simulink model "simModel"  (R2020a)
settings: Solver=VariableStepAuto  StartTime=0.0  StopTime=Simulation_Time  RelTol=1e-3
InitFcn:
  | ks = 500.4;
  | bs = 24.67;
  | 
  | ms = 325;               % 1/4 sprung mass (kg)
  | mus = 65;               % 1/4 unsprung mass (kg)
  | kus = 500.5e2;          % tire stiffness (N/m)
  | bus = 0;
  | grav = 9.81;            % acceleration of gravity (m/s^2)
  | v = 10;                 % vehicle velocity (m/s)
  | ts = 0.05;             % sampling time step
  | 
  | % Construct linear state space model
  | Aqcar = [-bs/ms -ks/ms bs/ms ks/ms;  1 0  0 0; bs/mus ks/mus -(bs+bus)/mus -(ks+kus)/mus; 0 0 1 0];
  | Bqcar = [1/ms 0 -1/mus 0;0 0 kus/mus 0]';
  | Cqcar = eye(4);
  | Dqcar = zeros(2,4)';
StopFcn:
  | clear ks bs  ms mus kus bus Aqcar Bqcar Cqcar Dqcar
values from neighbouring files (symbols this model uses):
  A = J    [CalculateMPC.m]    (also in CalculateMPC_IMP.m; Plant_Model.m = [ 0 0 1 0; returnStateSpace.m = [0 0 1 0)
  Aq = (eye(dimA)+A*T)    [FORWARDEULER.m]    (also in Get_Model_Script.m = [RP1.Data(end,[1:4]); Plant_Model_ZOH.m = sys.A)
  B = [0 0 ... (first row only)    [Plant_Model.m]    (also in returnStateSpace.m = [ 0 0 0)
  Bq = B*T    [FORWARDEULER.m]    (also in Get_Model_Script.m = [RP1.Data(end,[5:7]); Plant_Model_ZOH.m = sys.B)
  C = [-1 1 0 0 ... (first row only)    [Plant_Model.m]    (also in returnStateSpace.m)
  Cq = C    [FORWARDEULER.m]    (also in Plant_Model_ZOH.m = sys.C)
  D = [0 0;0 0; 0 -1; 0 0]    [Plant_Model.m]    (also in returnStateSpace.m = [0 0 0)
  Dq = D    [FORWARDEULER.m]    (also in Plant_Model_ZOH.m = sys.D)
  FILTER = 20    [BasicLeastSquares7.m]    (also in Get_Model_Script.m = 99999)
  NOISE = 0.00    (= 0)    [BasicLeastSquares7.m]    (also in BasicLeastSquares7_orig.m; CalculateMPC.m = 0.05; CalculateMPC_IMP.m = 0.05; Get_Model_Script.m = 0.05)
  SEED = 100    [Get_Model_Script.m]
  Simulation_Time = (points)*T    (= 100)    [BasicLeastSquares7.m]    (also in BasicLeastSquares7_orig.m = 10; Get_Model_Script.m = 500)
  T = 0.1    [BasicLeastSquares7.m]    (also in BasicLeastSquares7_orig.m = 0.0001; CalculateMPC.m = 0.05; CalculateMPC_IMP.m = 0.05; Get_Model_Script.m = 0.05)
libraries: simulink x7, cstblocks x1
PauseFcn:
  | clear ks bs  ms mus bus kus Aqcar Bqcar Cqcar Dqcar
settings Model: TunableVars=ts  TunableVarsStorageClass=Auto  Creator=manziec  LastModifiedBy=jakelangton
settings DataIOCC: SaveOutput=off  SaveTime=off  ReturnWorkspaceOutputs=off
settings OptimizationCC: DefaultParameterBehavior=Inlined
settings DebuggingCC: ArithmeticOperatorsInVariantConditions=warning
settings SFSimCC: CustomCodeUndefinedFunction=UseInterfaceOnly

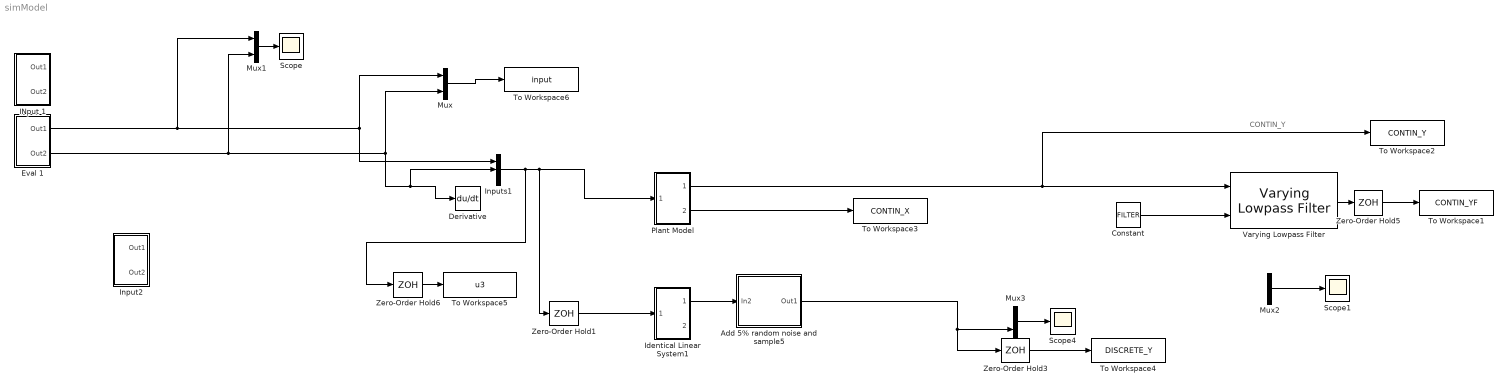
== system simModel ==
  note: CONTIN_Y
  Add 5% random noise and sample5 : Subsystem
  Constant : Constant  Value=FILTER
  Derivative : Derivative
  Eval 1 : Subsystem
  INput 1 : Subsystem
  Identical Linear System1 : Subsystem
  Input2 : Subsystem
  Inputs1 : Mux  Inputs=3
  Mux{,1..3} (4 alike) : Mux  Inputs=2
  Plant Model : Subsystem
  Scope : Scope
  Scope1 : Scope
  Scope4 : Scope
  To Workspace1 : ToWorkspace  VariableName=CONTIN_YF  SaveFormat=Timeseries  SampleTime=-1
  To Workspace2 : ToWorkspace  VariableName=CONTIN_Y  SaveFormat=Timeseries  SampleTime=-1
  To Workspace3 : ToWorkspace  VariableName=CONTIN_X  SaveFormat=Timeseries  SampleTime=-1
  To Workspace4 : ToWorkspace  VariableName=DISCRETE_Y  SaveFormat=Timeseries  SampleTime=-1
  To Workspace5 : ToWorkspace  VariableName=u3  SaveFormat=Timeseries  SampleTime=-1
  To Workspace6 : ToWorkspace  VariableName=input  SaveFormat=Timeseries  SampleTime=-1
  Varying Lowpass Filter : cstblocks/Linear Parameter Varying/Varying Lowpass Filter  N=1
  Zero-Order Hold{1,3,5..6} (4 alike) : ZeroOrderHold  SampleTime=T
  wires:
  Mux3/1 -> Scope4/1
  Inputs1/1 -> Zero-Order Hold6/1, Plant Model/1(In1), Zero-Order Hold1/1
  Add 5% random noise and sample5/1(Out1) -> Zero-Order Hold3/1, Mux3/2
  Identical Linear System1/1(Out1) -> Add 5% random noise and sample5/1(In2)
  Zero-Order Hold3/1 -> To Workspace4/1
  Zero-Order Hold6/1 -> To Workspace5/1
  Mux2/1 -> Scope1/1
  Zero-Order Hold1/1 -> Identical Linear System1/1(In1)
  Constant/1 -> Varying Lowpass Filter/2
  Zero-Order Hold5/1 -> To Workspace1/1
  Varying Lowpass Filter/1 -> Zero-Order Hold5/1
  Plant Model/1(Out1) -> To Workspace2/1, Varying Lowpass Filter/1
  Plant Model/2(Out2) -> To Workspace3/1
  Mux/1 -> To Workspace6/1
  Eval 1/2(Out2) -> Mux1/2, Derivative/1, Inputs1/2, Mux/2
  Mux1/1 -> Scope/1
  Eval 1/1(Out1) -> Mux1/1, Mux/1, Inputs1/1

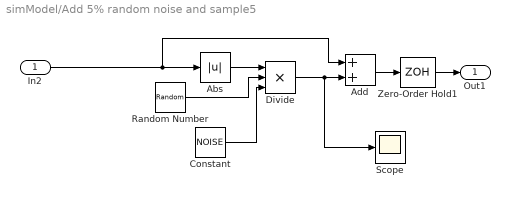
== system simModel/Add 5% random noise and sample5 ==
  In2 : Inport
  Abs : Abs
  Add : Sum
  Constant : Constant  Value=NOISE
  Divide : Product  Inputs=***
  Random Number : RandomNumber  Seed=123  SampleTime=T/10
  Scope : Scope
  Zero-Order Hold1 : ZeroOrderHold  SampleTime=T/10
  Out1 : Outport  VectorParamsAs1DForOutWhenUnconnected=off
  wires:
  Add/1 -> Zero-Order Hold1/1
  Zero-Order Hold1/1 -> Out1/1
  Random Number/1 -> Divide/2
  Abs/1 -> Divide/1
  In2/1 -> Abs/1, Add/1
  Constant/1 -> Divide/3
  Divide/1 -> Add/2, Scope/1

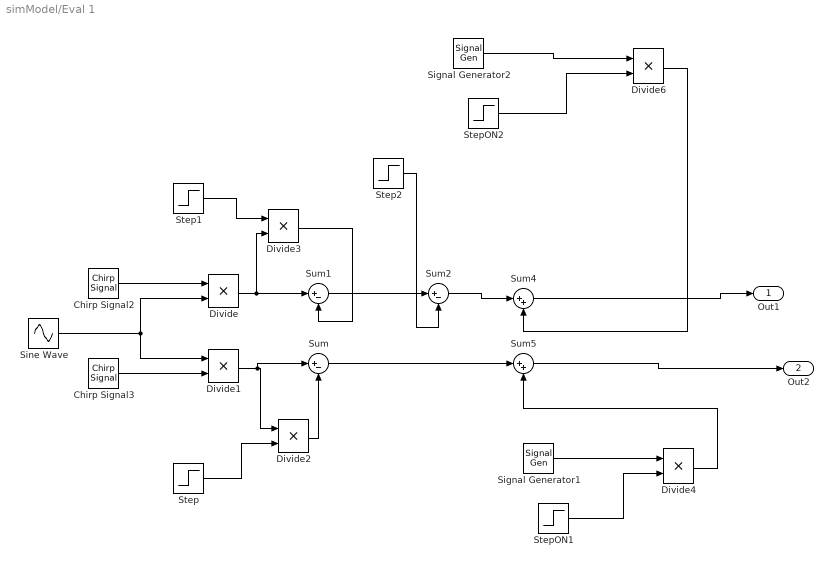
== system simModel/Eval 1 ==
  Chirp Signal2 : simulink/Sources/Chirp Signal  f1=0.01  T=Simulation_Time*3/4  f2=10
  Chirp Signal3 : simulink/Sources/Chirp Signal  f1=0.01  T=Simulation_Time*3/4  f2=5
  Divide{,1..4,6} (6 alike) : Product  Inputs=**
  Signal Generator1 : SignalGenerator  WaveForm=sawtooth  Frequency=4  Units=rad/sec
  Signal Generator2 : SignalGenerator  WaveForm=sawtooth  Frequency=7  Units=rad/sec
  Sine Wave : Sin  Amplitude=5  Frequency=0.5  SampleTime=0
  Step : Step  Time=Simulation_Time/2  SampleTime=0
  Step1 : Step  Time=Simulation_Time/2  SampleTime=0
  Step2 : Step  Time=Simulation_Time*3/5  SampleTime=0
  StepON1 : Step  Time=Simulation_Time*3/4  SampleTime=0
  StepON2 : Step  Time=Simulation_Time*3/4  SampleTime=0
  Sum : Sum  Inputs=|+-
  Sum1 : Sum  Inputs=|+-
  Sum2 : Sum  Inputs=|+-
  Sum4 : Sum  Inputs=|++
  Sum5 : Sum  Inputs=|++
  Out1 : Outport
  Out2 : Outport  Port=2
  wires:
  Sine Wave/1 -> Divide1/1, Divide/2
  Chirp Signal3/1 -> Divide1/2
  Step1/1 -> Divide3/1
  Chirp Signal2/1 -> Divide/1
  Divide/1 -> Divide3/2, Sum1/1
  Divide3/1 -> Sum1/2
  Step/1 -> Divide2/2
  Divide2/1 -> Sum/2
  Sum1/1 -> Sum2/1
  Divide1/1 -> Sum/1, Divide2/1
  Step2/1 -> Sum2/2
  StepON2/1 -> Divide6/2
  Signal Generator2/1 -> Divide6/1
  Sum2/1 -> Sum4/1
  Divide6/1 -> Sum4/2
  Sum/1 -> Sum5/1
  StepON1/1 -> Divide4/2
  Signal Generator1/1 -> Divide4/1
  Divide4/1 -> Sum5/2
  Sum4/1 -> Out1/1
  Sum5/1 -> Out2/1

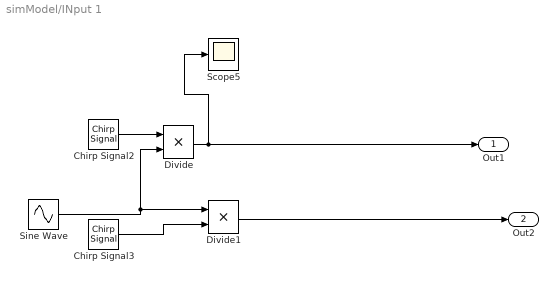
== system simModel/INput 1 ==
  Chirp Signal2 : simulink/Sources/Chirp Signal  f1=0.01  T=Simulation_Time  f2=10
  Chirp Signal3 : simulink/Sources/Chirp Signal  f1=0.01  T=Simulation_Time  f2=1
  Divide : Product  Inputs=**
  Divide1 : Product  Inputs=**
  Scope5 : Scope
  Sine Wave : Sin  Amplitude=10  Frequency=0.5  SampleTime=0
  Out1 : Outport
  Out2 : Outport  Port=2
  wires:
  Divide1/1 -> Out2/1
  Chirp Signal3/1 -> Divide1/2
  Divide/1 -> Out1/1, Scope5/1
  Chirp Signal2/1 -> Divide/1
  Sine Wave/1 -> Divide/2, Divide1/1

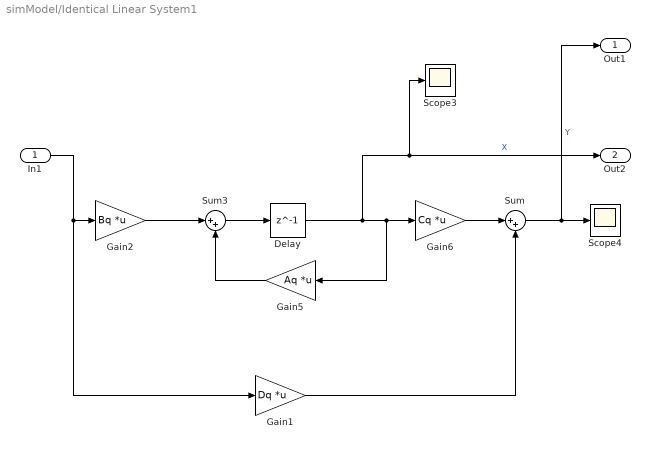
== system simModel/Identical Linear System1 ==
  In1 : Inport
  Delay : Delay  DelayLength=1
  Gain1 : Gain  Gain=Dq  Multiplication=Matrix(K*u)
  Gain2 : Gain  Gain=Bq  Multiplication=Matrix(K*u)
  Gain5 : Gain  Gain=Aq  Multiplication=Matrix(K*u)
  Gain6 : Gain  Gain=Cq  Multiplication=Matrix(K*u)
  Scope3 : Scope
  Scope4 : Scope
  Sum : Sum  Inputs=|++
  Sum3 : Sum  Inputs=|++
  Out1 : Outport
  Out2 : Outport  Port=2
  wires:
  Gain5/1 -> Sum3/2
  Sum3/1 -> Delay/1
  In1/1 -> Gain1/1, Gain2/1
  Delay/1 -> Scope3/1, Out2/1, Gain5/1, Gain6/1  "X"
  Gain6/1 -> Sum/1
  Sum/1 -> Out1/1, Scope4/1  "Y"
  Gain2/1 -> Sum3/1
  Gain1/1 -> Sum/2

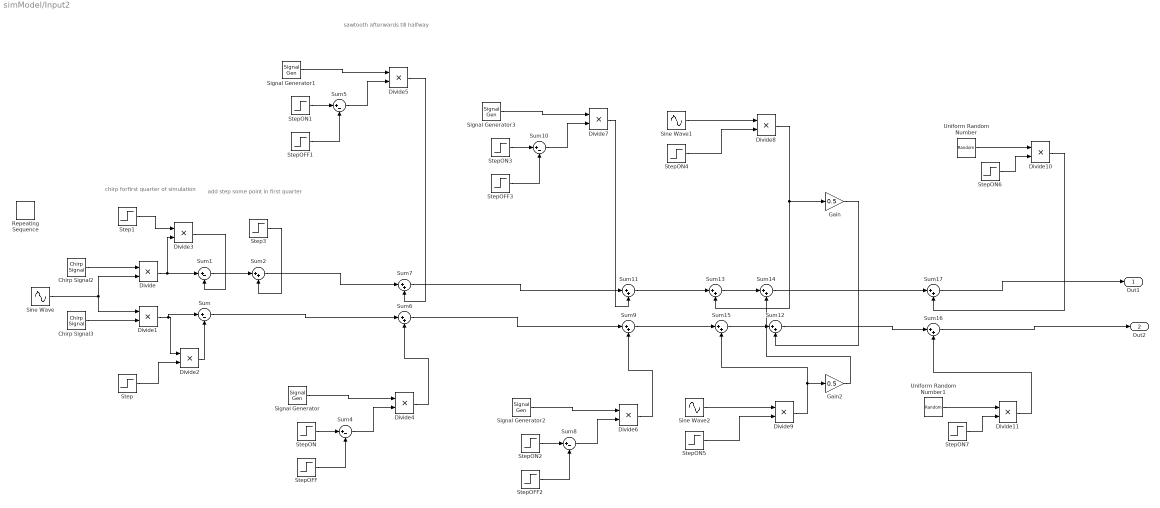
== system simModel/Input2 ==
  note: sawtooth afterwards till halfway
  note: add step some point in first quarter
  note: chirp forfirst quarter of simulation
  Chirp Signal2 : simulink/Sources/Chirp Signal  f1=0.01  T=Simulation_Time/4  f2=2
  Chirp Signal3 : simulink/Sources/Chirp Signal  f1=0.01  T=Simulation_Time/4  f2=1
  Divide{,1..11} (12 alike) : Product  Inputs=**
  Gain : Gain  Gain=0.5
  Gain2 : Gain  Gain=0.5
  Repeating Sequence : simulink/Sources/Repeating Sequence  rep_seq_t=[0 2]  rep_seq_y=[0 2]
  Signal Generator : SignalGenerator  WaveForm=sawtooth  Frequency=0.5  Units=rad/sec
  Signal Generator1 : SignalGenerator  WaveForm=sawtooth  Units=rad/sec
  Signal Generator2 : SignalGenerator  WaveForm=sawtooth  Frequency=0.02  Units=rad/sec
  Signal Generator3 : SignalGenerator  WaveForm=square  Frequency=0.1  Units=rad/sec
  Sine Wave : Sin  Amplitude=5  Frequency=0.5  SampleTime=0
  Sine Wave1 : Sin  SampleTime=0
  Sine Wave2 : Sin  SampleTime=0
  Step : Step  Time=Simulation_Time/4  SampleTime=0
  Step1 : Step  Time=Simulation_Time/4  SampleTime=0
  Step3 : Step  Before=10  SampleTime=0
  StepOFF : Step  Time=Simulation_Time/2  SampleTime=0
  StepOFF1 : Step  Time=Simulation_Time/2  SampleTime=0
  StepOFF2 : Step  Time=Simulation_Time/4 + Simulation_Time/2  SampleTime=0
  StepOFF3 : Step  Time=Simulation_Time/2 + Simulation_Time/3  SampleTime=0
  StepON : Step  Time=Simulation_Time/4 + Simulation_Time/12  SampleTime=0
  StepON1 : Step  Time=Simulation_Time/4 + Simulation_Time/16  SampleTime=0
  StepON2 : Step  Time=Simulation_Time/4 + Simulation_Time/8  SampleTime=0
  StepON3 : Step  Time=Simulation_Time/4 + Simulation_Time/7  SampleTime=0
  StepON4 : Step  Time=Simulation_Time/2 + Simulation_Time/4  SampleTime=0
  StepON5 : Step  Time=Simulation_Time/2 + Simulation_Time/6  After=2  SampleTime=0
  StepON6 : Step  Time=Simulation_Time/2 + Simulation_Time/2.8  SampleTime=0
  StepON7 : Step  Time=Simulation_Time/2 + Simulation_Time/3.1  SampleTime=0
  Sum{,1,4..5,8,10} (6 alike) : Sum  Inputs=|+-
  Sum{2,6..7,9,11..17} (11 alike) : Sum  Inputs=|++
  Uniform Random Number : UniformRandomNumber  Minimum=-0.2  Maximum=0.2  SampleTime=0.1
  Uniform Random Number1 : UniformRandomNumber  Minimum=-0.2  Maximum=0.2  SampleTime=0.1
  Out1 : Outport
  Out2 : Outport  Port=2
  wires:
  Chirp Signal3/1 -> Divide1/2
  Sine Wave/1 -> Divide1/1, Divide/2
  Chirp Signal2/1 -> Divide/1
  Divide/1 -> Divide3/2, Sum1/1
  Step/1 -> Divide2/2
  Divide1/1 -> Sum/1, Divide2/1
  Divide2/1 -> Sum/2
  Divide3/1 -> Sum1/2
  Step1/1 -> Divide3/1
  Sum1/1 -> Sum2/1
  Step3/1 -> Sum2/2
  Signal Generator/1 -> Divide4/1
  StepON/1 -> Sum4/1
  StepOFF/1 -> Sum4/2
  Sum4/1 -> Divide4/2
  Signal Generator1/1 -> Divide5/1
  Sum5/1 -> Divide5/2
  StepOFF1/1 -> Sum5/2
  StepON1/1 -> Sum5/1
  Sum/1 -> Sum6/1
  Sum2/1 -> Sum7/1
  Divide5/1 -> Sum7/2
  Divide4/1 -> Sum6/2
  Signal Generator2/1 -> Divide6/1
  Sum8/1 -> Divide6/2
  StepOFF2/1 -> Sum8/2
  StepON2/1 -> Sum8/1
  Divide6/1 -> Sum9/2
  Sum6/1 -> Sum9/1
  Divide7/1 -> Sum11/2
  StepOFF3/1 -> Sum10/2
  StepON3/1 -> Sum10/1
  Signal Generator3/1 -> Divide7/1
  Sum10/1 -> Divide7/2
  Sum7/1 -> Sum11/1
  StepON4/1 -> Divide8/2
  Sine Wave1/1 -> Divide8/1
  Sum11/1 -> Sum13/1
  Divide8/1 -> Gain/1, Sum13/2
  StepON5/1 -> Divide9/2
  Sine Wave2/1 -> Divide9/1
  Divide9/1 -> Gain2/1, Sum15/2
  Sum9/1 -> Sum15/1
  Sum15/1 -> Sum12/1
  Gain/1 -> Sum12/2
  Gain2/1 -> Sum14/2
  Sum13/1 -> Sum14/1
  Uniform Random Number/1 -> Divide10/1
  StepON6/1 -> Divide10/2
  Uniform Random Number1/1 -> Divide11/1
  StepON7/1 -> Divide11/2
  Sum12/1 -> Sum16/1
  Sum14/1 -> Sum17/1
  Divide10/1 -> Sum17/2
  Divide11/1 -> Sum16/2
  Sum17/1 -> Out1/1
  Sum16/1 -> Out2/1

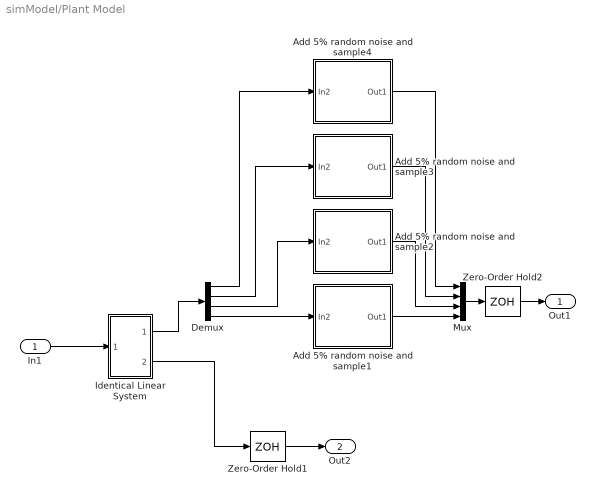
== system simModel/Plant Model ==
  In1 : Inport
  Add 5% random noise and sample1 : Subsystem
  Add 5% random noise and sample2 : Subsystem
  Add 5% random noise and sample3 : Subsystem
  Add 5% random noise and sample4 : Subsystem
  Demux : Demux
  Identical Linear System : Subsystem
  Mux : Mux
  Zero-Order Hold1 : ZeroOrderHold  SampleTime=T
  Zero-Order Hold2 : ZeroOrderHold  SampleTime=T
  Out1 : Outport
  Out2 : Outport  Port=2
  wires:
  In1/1 -> Identical Linear System/1(In1)
  Zero-Order Hold2/1 -> Out1/1
  Mux/1 -> Zero-Order Hold2/1
  Add 5% random noise and sample4/1(Out1) -> Mux/1
  Add 5% random noise and sample3/1(Out1) -> Mux/2
  Add 5% random noise and sample2/1(Out1) -> Mux/3
  Add 5% random noise and sample1/1(Out1) -> Mux/4
  Demux/4 -> Add 5% random noise and sample1/1(In2)
  Demux/3 -> Add 5% random noise and sample2/1(In2)
  Demux/2 -> Add 5% random noise and sample3/1(In2)
  Demux/1 -> Add 5% random noise and sample4/1(In2)
  Identical Linear System/1(Out1) -> Demux/1
  Zero-Order Hold1/1 -> Out2/1
  Identical Linear System/2(Out2) -> Zero-Order Hold1/1

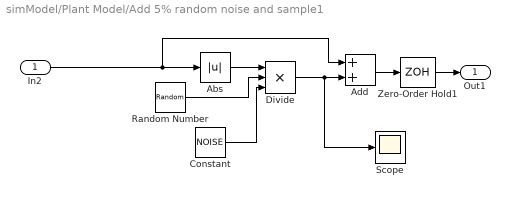
== system simModel/Plant Model/Add 5% random noise and sample1 ==
  In2 : Inport
  Abs : Abs
  Add : Sum
  Constant : Constant  Value=NOISE
  Divide : Product  Inputs=***
  Random Number : RandomNumber  Seed=SEED+103  SampleTime=T/10
  Scope : Scope
  Zero-Order Hold1 : ZeroOrderHold  SampleTime=T/10
  Out1 : Outport  VectorParamsAs1DForOutWhenUnconnected=off
  wires:
  Add/1 -> Zero-Order Hold1/1
  Zero-Order Hold1/1 -> Out1/1
  Random Number/1 -> Divide/2
  Abs/1 -> Divide/1
  In2/1 -> Abs/1, Add/1
  Constant/1 -> Divide/3
  Divide/1 -> Add/2, Scope/1

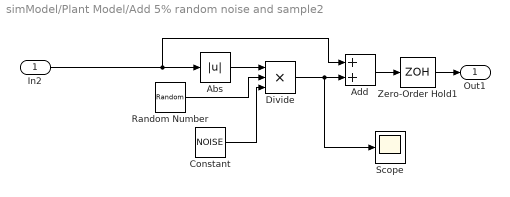
== system simModel/Plant Model/Add 5% random noise and sample2 ==
  In2 : Inport
  Abs : Abs
  Add : Sum
  Constant : Constant  Value=NOISE
  Divide : Product  Inputs=***
  Random Number : RandomNumber  Seed=SEED+102  SampleTime=T/10
  Scope : Scope
  Zero-Order Hold1 : ZeroOrderHold  SampleTime=T/10
  Out1 : Outport  VectorParamsAs1DForOutWhenUnconnected=off
  wires:
  Add/1 -> Zero-Order Hold1/1
  Zero-Order Hold1/1 -> Out1/1
  Random Number/1 -> Divide/2
  Abs/1 -> Divide/1
  In2/1 -> Abs/1, Add/1
  Constant/1 -> Divide/3
  Divide/1 -> Add/2, Scope/1

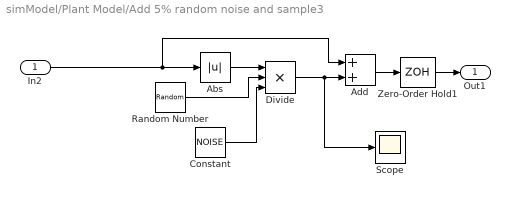
== system simModel/Plant Model/Add 5% random noise and sample3 ==
  In2 : Inport
  Abs : Abs
  Add : Sum
  Constant : Constant  Value=NOISE
  Divide : Product  Inputs=***
  Random Number : RandomNumber  Seed=SEED+101  SampleTime=T/10
  Scope : Scope
  Zero-Order Hold1 : ZeroOrderHold  SampleTime=T/10
  Out1 : Outport  VectorParamsAs1DForOutWhenUnconnected=off
  wires:
  Add/1 -> Zero-Order Hold1/1
  Zero-Order Hold1/1 -> Out1/1
  Random Number/1 -> Divide/2
  Abs/1 -> Divide/1
  In2/1 -> Abs/1, Add/1
  Constant/1 -> Divide/3
  Divide/1 -> Add/2, Scope/1

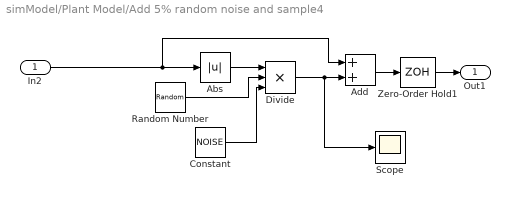
== system simModel/Plant Model/Add 5% random noise and sample4 ==
  In2 : Inport
  Abs : Abs
  Add : Sum
  Constant : Constant  Value=NOISE
  Divide : Product  Inputs=***
  Random Number : RandomNumber  Seed=SEED+100  SampleTime=T/10
  Scope : Scope
  Zero-Order Hold1 : ZeroOrderHold  SampleTime=T/10
  Out1 : Outport  VectorParamsAs1DForOutWhenUnconnected=off
  wires:
  Add/1 -> Zero-Order Hold1/1
  Zero-Order Hold1/1 -> Out1/1
  Random Number/1 -> Divide/2
  Abs/1 -> Divide/1
  In2/1 -> Abs/1, Add/1
  Constant/1 -> Divide/3
  Divide/1 -> Add/2, Scope/1

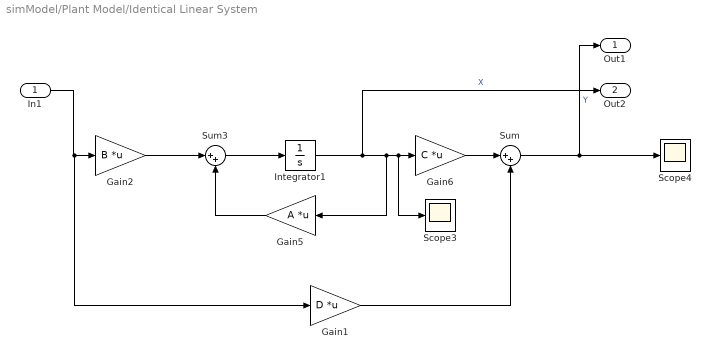
== system simModel/Plant Model/Identical Linear System ==
  In1 : Inport
  Gain1 : Gain  Gain=D  Multiplication=Matrix(K*u)
  Gain2 : Gain  Gain=B  Multiplication=Matrix(K*u)
  Gain5 : Gain  Gain=A  Multiplication=Matrix(K*u)
  Gain6 : Gain  Gain=C  Multiplication=Matrix(K*u)
  Integrator1 : Integrator
  Scope3 : Scope
  Scope4 : Scope
  Sum : Sum  Inputs=|++
  Sum3 : Sum  Inputs=|++
  Out1 : Outport
  Out2 : Outport  Port=2
  wires:
  Gain5/1 -> Sum3/2
  Sum3/1 -> Integrator1/1
  In1/1 -> Gain1/1, Gain2/1
  Gain2/1 -> Sum3/1
  Integrator1/1 -> Out2/1, Gain5/1, Scope3/1, Gain6/1  "X"
  Gain6/1 -> Sum/1
  Sum/1 -> Out1/1, Scope4/1  "Y"
  Gain1/1 -> Sum/2
